simulink library "halout"  (R2021b)
settings: Solver=VariableStepAuto  StartTime=0.0  StopTime=10.0  RelTol=1e-3
undefined symbols (not defined in the file): C_TASK_5MS_S, FALSE, KHAL_CAN1TxReq_flg, KHAL_CAN2TxReq_flg, KHAL_CAN3FD3VCU1toNIDECTxReq_flg, KHAL_CAN3FD3VCU1TxReq_flg, KHAL_CAN3FD3VCU2E2E_flg, KHAL_CAN3FD3VCU2toNIDECE2E_flg, KHAL_CAN3FD3VCU2toNIDECTxReq_flg, KHAL_CAN3FD3VCU2TxReq_flg, KHAL_CAN3TxReq_flg, KHAL_CAN4FD4CE1000E2E_flg, KHAL_CAN4FD4CE1000TxReq_flg, KHAL_CAN4TxReq_flg, KHAL_CAN5TxReq_flg, KHAL_CAN7TxReq_flg, ONE_INT, TRUE, ZERO_INT
libraries: FVT_lib x258, simulink x115
(part 8 of 17)

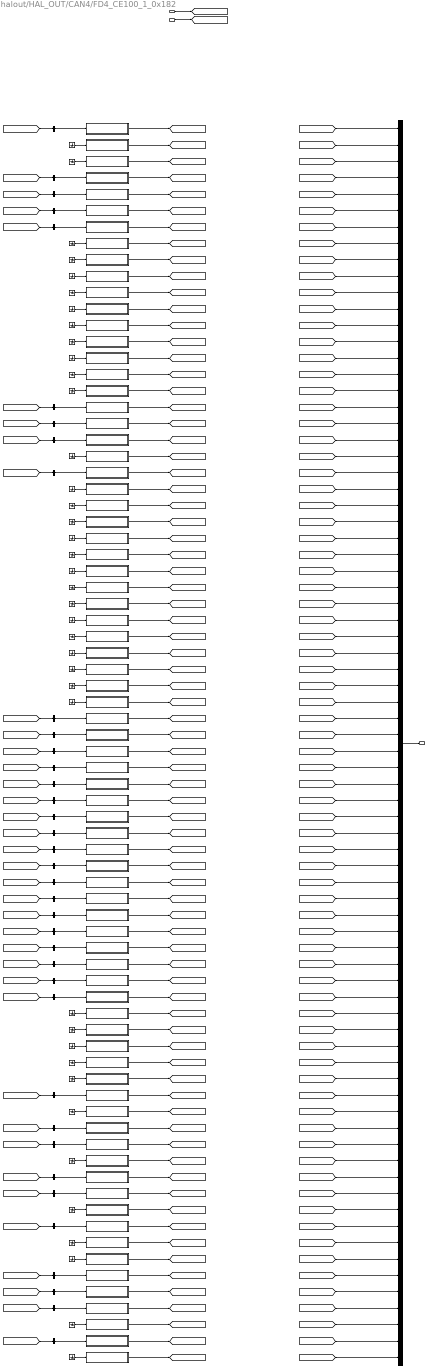
== system halout/HAL_OUT/CAN4/FD4_CE100_1_0x182 ==
  BSCP_outputs : Inport  OutDataTypeStr=Bus: BSCP_outputs
  BOUTP_outputs : Inport  Port=2  OutDataTypeStr=Bus: BOUTP_outputs
  ACSubMode : Subsystem
  APTCActFrRiPwr : Subsystem
  BatLoopActWtFlw : Subsystem
  BatteryMode : Subsystem
  CCUACLampSts : Subsystem
  CCUACMaxLampSts : Subsystem
  CCUAutoLampSts : Subsystem
  CCUAutoMidLampSts : Subsystem
  CCUCbnPreACWkSts : Subsystem
  CCUCbnPreEstimdTi : Subsystem
  CCUCbnPreSts : Subsystem
  CCUDispalyRequest : Subsystem
  CCUEcoSts : Subsystem
  CCUFrtOnOffLampSts : Subsystem
  CCUHEATMaxLampSts : Subsystem
  CCUHiVoltageReq : Subsystem
  CCURrOnOffLampSts : Subsystem
  CCUSyncLampSts : Subsystem
  CabinMode : Subsystem
  CoolgFanActDuty : Subsystem
  DeiceModReq : Subsystem
  EDriveMode : Subsystem
  FDBlowerCmd : Subsystem
  FDCTHCMCLEVentYSta : Subsystem
  FDCTHCMCLEVentZSta : Subsystem
  FDCTHCMCLVentSta : Subsystem
  FDCTHCMCREVentYSta : Subsystem
  FDCTHCMCREVentZSta : Subsystem
  FDCTHCMCRVentSta : Subsystem
  FDCTHCMDrEVentModeSta : Subsystem
  FDCTHCMDrEVentYSta : Subsystem
  FDCTHCMDrEVentZSta : Subsystem
  FDCTHCMDrVentSta : Subsystem
  FDCTHCMPsEVentModeSta : Subsystem
  FDCTHCMPsEVentYSta : Subsystem
  FDCTHCMPsEVentZSta : Subsystem
  FDCTHCMPsVentSta : Subsystem
  FDCompCmd : Subsystem
  FDEWP1Cmd : Subsystem
  FDEWP2Cmd : Subsystem
  FDEWP3Cmd : Subsystem
  FDEXV1Cmd : Subsystem
  FDEXV2Cmd : Subsystem
  FDFWVCmd : Subsystem
  FDFrLeAPTCHeatPwrCmd : Subsystem
  FDFrRiAPTCHeatPwrCmd : Subsystem
  FDFrWPTCHeatPwrCmd : Subsystem
  FDRecyAutoCmd : Subsystem
  FDRrAPTCHeatPwrCmd : Subsystem
  FDSOTXVCmd : Subsystem
  FDSOV1Cmd : Subsystem
  FDSOV2Cmd : Subsystem
  FDSOV3Cmd : Subsystem
  FDTWVCmd : Subsystem
  FrCoolantflow : Subsystem
  FrCoolanttemp : Subsystem
  Ground{,1..38} (39 alike) : Ground
  HPThermalRecoveryReq : Subsystem
  RrCoolantflow : Subsystem
  RrCoolanttemp : Subsystem
  bus_creator : BusCreator  Inputs=76  OutDataTypeStr=Bus: DT_CAN4_SG_FD4_CE100_1  NonVirtualBus=on
  bus_selector : BusSelector  OutputSignals=VOUTP_ACSubMode_enum
  bus_selector1 : BusSelector  OutputSignals=VOUTP_BatteryMode_enum
  bus_selector10 : BusSelector  OutputSignals=VOUTP_FDCompCmd_rpm
  bus_selector11 : BusSelector  OutputSignals=VOUTP_FDEWP1Cmd_enum
  bus_selector12 : BusSelector  OutputSignals=VOUTP_FDEWP2Cmd_enum
  bus_selector13 : BusSelector  OutputSignals=VOUTP_FDEWP3Cmd_enum
  bus_selector14 : BusSelector  OutputSignals=VOUTP_FDEXV1Cmd_step
  bus_selector15 : BusSelector  OutputSignals=VOUTP_FDEXV2Cmd_step
  bus_selector16 : BusSelector  OutputSignals=VOUTP_FDFWVCmd_flg
  bus_selector17 : BusSelector  OutputSignals=VOUTP_FDFrLeAPTCHeatPwrCmd_W
  bus_selector18 : BusSelector  OutputSignals=VOUTP_FDFrRiAPTCHeatPwrCmd_W
  bus_selector19 : BusSelector  OutputSignals=VOUTP_FDFrWPTCHeatPwrCmd_W
  bus_selector2 : BusSelector  OutputSignals=VOUTP_CCUACLampSts_flg
  bus_selector20 : BusSelector  OutputSignals=VOUTP_FDRecyAutoCmd_enum
  bus_selector21 : BusSelector  OutputSignals=VOUTP_FDRrAPTCHeatPwrCmd_W
  bus_selector22 : BusSelector  OutputSignals=VOUTP_FDSOTXVCmd_flg
  bus_selector23 : BusSelector  OutputSignals=VOUTP_FDSOV1Cmd_flg
  bus_selector24 : BusSelector  OutputSignals=VOUTP_FDSOV2Cmd_flg
  bus_selector25 : BusSelector  OutputSignals=VOUTP_FDSOV3Cmd_flg
  bus_selector26 : BusSelector  OutputSignals=VOUTP_FDTWVCmd_pct
  bus_selector27 : BusSelector  OutputSignals=VOUTP_sigAirIntenZon1St_enum
  bus_selector28 : BusSelector  OutputSignals=VOUTP_sigAmbAirT_C
  bus_selector29 : BusSelector  OutputSignals=VOUTP_sigCbnAirT_C
  bus_selector3 : BusSelector  OutputSignals=VOUTP_CCUACMaxLampSts_flg
  bus_selector30 : BusSelector  OutputSignals=VOUTP_sigCbnSolarLeft_W
  bus_selector31 : BusSelector  OutputSignals=VOUTP_sigCbnSolarRight_W
  bus_selector32 : BusSelector  OutputSignals=VOUTP_sigClntTHvBattOut_C
  bus_selector33 : BusSelector  OutputSignals=VOUTP_sigRecircSt_flg
  bus_selector34 : BusSelector  OutputSignals=VOUTP_sigSetTempZon1St_C
  bus_selector35 : BusSelector  OutputSignals=VOUTP_sigSetTempZon2St_C
  bus_selector36 : BusSelector  OutputSignals=VOUTP_sigWindDirZon1St_enum
  bus_selector4 : BusSelector  OutputSignals=VOUTP_CCUAutoLampSts_flg
  bus_selector5 : BusSelector  OutputSignals=VOUTP_CCUSyncLampSts_flg
  bus_selector6 : BusSelector  OutputSignals=VOUTP_CabinMode_enum
  bus_selector7 : BusSelector  OutputSignals=VOUTP_CoolgFanActDuty_pct
  bus_selector8 : BusSelector  OutputSignals=VOUTP_EDriveMode_enum
  bus_selector9 : BusSelector  OutputSignals=VOUTP_FDBlowerCmd_pct
  sigAirIntenZon1St : Subsystem
  sigAirIntenZon3St : Subsystem
  sigAmbAirT : Subsystem
  sigCbnAirT : Subsystem
  sigCbnPTCPwrAct : Subsystem
  sigCbnSolarLeft : Subsystem
  sigCbnSolarRight : Subsystem
  sigClmtCmprPwrAct : Subsystem
  sigClntTHvBattOut : Subsystem
  sigDfrstSt : Subsystem
  sigHvacSt : Subsystem
  sigRecircSt : Subsystem
  sigSetTempZon1St : Subsystem
  sigSetTempZon2St : Subsystem
  sigSetTempZon3St : Subsystem
  sigWindDirZon1St : Subsystem
  sigWindDirZon3St : Subsystem
  FD4_CE100_1 : Outport
  wires:
  BSCP_outputs/1 -> [BSCP_outputs]
  BOUTP_outputs/1 -> [BOUTP_outputs]
  [CAN4_ACSubMode] -> bus_creator/1  "CAN4_ACSubMode"
  [CAN4_APTC_ActFrRiPwr] -> bus_creator/2  "CAN4_APTC_ActFrRiPwr"
  [CAN4_BatLoopActWtFlw] -> bus_creator/3  "CAN4_BatLoopActWtFlw"
  [CAN4_BatteryMode] -> bus_creator/4  "CAN4_BatteryMode"
  [CAN4_CCU_ACLampSts] -> bus_creator/5  "CAN4_CCU_ACLampSts"
  [CAN4_CCU_ACMaxLampSts] -> bus_creator/6  "CAN4_CCU_ACMaxLampSts"
  [CAN4_CCU_AutoLampSts] -> bus_creator/7  "CAN4_CCU_AutoLampSts"
  [CAN4_CCU_AutoMidLampSts] -> bus_creator/8  "CAN4_CCU_AutoMidLampSts"
  [CAN4_CCU_CbnPreACWkSts] -> bus_creator/9  "CAN4_CCU_CbnPreACWkSts"
  [CAN4_CCU_CbnPreEstimdTi] -> bus_creator/10  "CAN4_CCU_CbnPreEstimdTi"
  [CAN4_CCU_CbnPreSts] -> bus_creator/11  "CAN4_CCU_CbnPreSts"
  [CAN4_CCU_Dispaly_Request] -> bus_creator/12  "CAN4_CCU_Dispaly_Request"
  [CAN4_CCU_EcoSts] -> bus_creator/13  "CAN4_CCU_EcoSts"
  [CAN4_CCU_FrtOnOffLampSts] -> bus_creator/14  "CAN4_CCU_FrtOnOffLampSts"
  [CAN4_CCU_HEATMaxLampSts] -> bus_creator/15  "CAN4_CCU_HEATMaxLampSts"
  [CAN4_CCU_HiVoltageReq] -> bus_creator/16  "CAN4_CCU_HiVoltageReq"
  [CAN4_CCU_RrOnOffLampSts] -> bus_creator/17  "CAN4_CCU_RrOnOffLampSts"
  [CAN4_CCU_SyncLampSts] -> bus_creator/18  "CAN4_CCU_SyncLampSts"
  [CAN4_CabinMode] -> bus_creator/19  "CAN4_CabinMode"
  [CAN4_CoolgFanActDuty] -> bus_creator/20  "CAN4_CoolgFanActDuty"
  [CAN4_DeiceModReq] -> bus_creator/21  "CAN4_DeiceModReq"
  [CAN4_EDriveMode] -> bus_creator/22  "CAN4_EDriveMode"
  [CAN4_FDC_THCM_CLEVentY_Sta] -> bus_creator/23  "CAN4_FDC_THCM_CLEVentY_Sta"
  [CAN4_FDC_THCM_CLEVentZ_Sta] -> bus_creator/24  "CAN4_FDC_THCM_CLEVentZ_Sta"
  [CAN4_FDC_THCM_CLVent_Sta] -> bus_creator/25  "CAN4_FDC_THCM_CLVent_Sta"
  [CAN4_FDC_THCM_CREVentY_Sta] -> bus_creator/26  "CAN4_FDC_THCM_CREVentY_Sta"
  [CAN4_FDC_THCM_CREVentZ_Sta] -> bus_creator/27  "CAN4_FDC_THCM_CREVentZ_Sta"
  [CAN4_FDC_THCM_CRVent_Sta] -> bus_creator/28  "CAN4_FDC_THCM_CRVent_Sta"
  [CAN4_FDC_THCM_DrEVentMode_Sta] -> bus_creator/29  "CAN4_FDC_THCM_DrEVentMode_Sta"
  [CAN4_FDC_THCM_DrEVentY_Sta] -> bus_creator/30  "CAN4_FDC_THCM_DrEVentY_Sta"
  [CAN4_FDC_THCM_DrEVentZ_Sta] -> bus_creator/31  "CAN4_FDC_THCM_DrEVentZ_Sta"
  [CAN4_FDC_THCM_DrVent_Sta] -> bus_creator/32  "CAN4_FDC_THCM_DrVent_Sta"
  [CAN4_FDC_THCM_PsEVentMode_Sta] -> bus_creator/33  "CAN4_FDC_THCM_PsEVentMode_Sta"
  [CAN4_FDC_THCM_PsEVentY_Sta] -> bus_creator/34  "CAN4_FDC_THCM_PsEVentY_Sta"
  [CAN4_FDC_THCM_PsEVentZ_Sta] -> bus_creator/35  "CAN4_FDC_THCM_PsEVentZ_Sta"
  [CAN4_FDC_THCM_PsVent_Sta] -> bus_creator/36  "CAN4_FDC_THCM_PsVent_Sta"
  [CAN4_FD_Blower_Cmd] -> bus_creator/37  "CAN4_FD_Blower_Cmd"
  [CAN4_FD_Comp_Cmd] -> bus_creator/38  "CAN4_FD_Comp_Cmd"
  [CAN4_FD_EWP1_Cmd] -> bus_creator/39  "CAN4_FD_EWP1_Cmd"
  [CAN4_FD_EWP2_Cmd] -> bus_creator/40  "CAN4_FD_EWP2_Cmd"
  [CAN4_FD_EWP3_Cmd] -> bus_creator/41  "CAN4_FD_EWP3_Cmd"
  [CAN4_FD_EXV1_Cmd] -> bus_creator/42  "CAN4_FD_EXV1_Cmd"
  [CAN4_FD_EXV2_Cmd] -> bus_creator/43  "CAN4_FD_EXV2_Cmd"
  [CAN4_FD_FWV_Cmd] -> bus_creator/44  "CAN4_FD_FWV_Cmd"
  [CAN4_FD_FrLeAPTCHeatPwr_Cmd] -> bus_creator/45  "CAN4_FD_FrLeAPTCHeatPwr_Cmd"
  [CAN4_FD_FrRiAPTCHeatPwr_Cmd] -> bus_creator/46  "CAN4_FD_FrRiAPTCHeatPwr_Cmd"
  [CAN4_FD_FrWPTCHeatPwr_Cmd] -> bus_creator/47  "CAN4_FD_FrWPTCHeatPwr_Cmd"
  [CAN4_FD_RecyAuto_Cmd] -> bus_creator/48  "CAN4_FD_RecyAuto_Cmd"
  [CAN4_FD_RrAPTCHeatPwr_Cmd] -> bus_creator/49  "CAN4_FD_RrAPTCHeatPwr_Cmd"
  [CAN4_FD_SOTXV_Cmd] -> bus_creator/50  "CAN4_FD_SOTXV_Cmd"
  [CAN4_FD_SOV1_Cmd] -> bus_creator/51  "CAN4_FD_SOV1_Cmd"
  [CAN4_FD_SOV2_Cmd] -> bus_creator/52  "CAN4_FD_SOV2_Cmd"
  [CAN4_FD_SOV3_Cmd] -> bus_creator/53  "CAN4_FD_SOV3_Cmd"
  [CAN4_FD_TWV_Cmd] -> bus_creator/54  "CAN4_FD_TWV_Cmd"
  [CAN4_Fr_Coolantflow] -> bus_creator/55  "CAN4_Fr_Coolantflow"
  [CAN4_Fr_Coolanttemp] -> bus_creator/56  "CAN4_Fr_Coolanttemp"
  [CAN4_HPThermalRecoveryReq] -> bus_creator/57  "CAN4_HPThermalRecoveryReq"
  [CAN4_Rr_Coolantflow] -> bus_creator/58  "CAN4_Rr_Coolantflow"
  [CAN4_Rr_Coolanttemp] -> bus_creator/59  "CAN4_Rr_Coolanttemp"
  [CAN4_sigAirIntenZon1St] -> bus_creator/60  "CAN4_sigAirIntenZon1St"
  [CAN4_sigAirIntenZon3St] -> bus_creator/61  "CAN4_sigAirIntenZon3St"
  [CAN4_sigAmbAirT] -> bus_creator/62  "CAN4_sigAmbAirT"
  [CAN4_sigCbnAirT] -> bus_creator/63  "CAN4_sigCbnAirT"
  [CAN4_sigCbnPTCPwrAct] -> bus_creator/64  "CAN4_sigCbnPTCPwrAct"
  [CAN4_sigCbnSolarLeft] -> bus_creator/65  "CAN4_sigCbnSolarLeft"
  [CAN4_sigCbnSolarRight] -> bus_creator/66  "CAN4_sigCbnSolarRight"
  [CAN4_sigClmtCmprPwrAct] -> bus_creator/67  "CAN4_sigClmtCmprPwrAct"
  [CAN4_sigClntTHvBattOut] -> bus_creator/68  "CAN4_sigClntTHvBattOut"
  [CAN4_sigDfrstSt] -> bus_creator/69  "CAN4_sigDfrstSt"
  [CAN4_sigHvacSt] -> bus_creator/70  "CAN4_sigHvacSt"
  [CAN4_sigRecircSt] -> bus_creator/71  "CAN4_sigRecircSt"
  [CAN4_sigSetTempZon1St] -> bus_creator/72  "CAN4_sigSetTempZon1St"
  [CAN4_sigSetTempZon2St] -> bus_creator/73  "CAN4_sigSetTempZon2St"
  [CAN4_sigSetTempZon3St] -> bus_creator/74  "CAN4_sigSetTempZon3St"
  [CAN4_sigWindDirZon1St] -> bus_creator/75  "CAN4_sigWindDirZon1St"
  [CAN4_sigWindDirZon3St] -> bus_creator/76  "CAN4_sigWindDirZon3St"
  bus_creator/1 -> FD4_CE100_1/1
  ACSubMode/1(CAN4_ACSubMode) -> [CAN4_ACSubMode]
  APTCActFrRiPwr/1(CAN4_APTC_ActFrRiPwr) -> [CAN4_APTC_ActFrRiPwr]
  BatLoopActWtFlw/1(CAN4_BatLoopActWtFlw) -> [CAN4_BatLoopActWtFlw]
  BatteryMode/1(CAN4_BatteryMode) -> [CAN4_BatteryMode]
  CCUACLampSts/1(CAN4_CCU_ACLampSts) -> [CAN4_CCU_ACLampSts]
  CCUACMaxLampSts/1(CAN4_CCU_ACMaxLampSts) -> [CAN4_CCU_ACMaxLampSts]
  CCUAutoLampSts/1(CAN4_CCU_AutoLampSts) -> [CAN4_CCU_AutoLampSts]
  CCUAutoMidLampSts/1(CAN4_CCU_AutoMidLampSts) -> [CAN4_CCU_AutoMidLampSts]
  CCUCbnPreACWkSts/1(CAN4_CCU_CbnPreACWkSts) -> [CAN4_CCU_CbnPreACWkSts]
  CCUCbnPreEstimdTi/1(CAN4_CCU_CbnPreEstimdTi) -> [CAN4_CCU_CbnPreEstimdTi]
  CCUCbnPreSts/1(CAN4_CCU_CbnPreSts) -> [CAN4_CCU_CbnPreSts]
  CCUDispalyRequest/1(CAN4_CCU_Dispaly_Request) -> [CAN4_CCU_Dispaly_Request]
  CCUEcoSts/1(CAN4_CCU_EcoSts) -> [CAN4_CCU_EcoSts]
  CCUFrtOnOffLampSts/1(CAN4_CCU_FrtOnOffLampSts) -> [CAN4_CCU_FrtOnOffLampSts]
  CCUHEATMaxLampSts/1(CAN4_CCU_HEATMaxLampSts) -> [CAN4_CCU_HEATMaxLampSts]
  CCUHiVoltageReq/1(CAN4_CCU_HiVoltageReq) -> [CAN4_CCU_HiVoltageReq]
  CCURrOnOffLampSts/1(CAN4_CCU_RrOnOffLampSts) -> [CAN4_CCU_RrOnOffLampSts]
  CCUSyncLampSts/1(CAN4_CCU_SyncLampSts) -> [CAN4_CCU_SyncLampSts]
  CabinMode/1(CAN4_CabinMode) -> [CAN4_CabinMode]
  CoolgFanActDuty/1(CAN4_CoolgFanActDuty) -> [CAN4_CoolgFanActDuty]
  DeiceModReq/1(CAN4_DeiceModReq) -> [CAN4_DeiceModReq]
  EDriveMode/1(CAN4_EDriveMode) -> [CAN4_EDriveMode]
  FDCTHCMCLEVentYSta/1(CAN4_FDC_THCM_CLEVentY_Sta) -> [CAN4_FDC_THCM_CLEVentY_Sta]
  FDCTHCMCLEVentZSta/1(CAN4_FDC_THCM_CLEVentZ_Sta) -> [CAN4_FDC_THCM_CLEVentZ_Sta]
  FDCTHCMCLVentSta/1(CAN4_FDC_THCM_CLVent_Sta) -> [CAN4_FDC_THCM_CLVent_Sta]
  FDCTHCMCREVentYSta/1(CAN4_FDC_THCM_CREVentY_Sta) -> [CAN4_FDC_THCM_CREVentY_Sta]
  FDCTHCMCREVentZSta/1(CAN4_FDC_THCM_CREVentZ_Sta) -> [CAN4_FDC_THCM_CREVentZ_Sta]
  FDCTHCMCRVentSta/1(CAN4_FDC_THCM_CRVent_Sta) -> [CAN4_FDC_THCM_CRVent_Sta]
  FDCTHCMDrEVentModeSta/1(CAN4_FDC_THCM_DrEVentMode_Sta) -> [CAN4_FDC_THCM_DrEVentMode_Sta]
  FDCTHCMDrEVentYSta/1(CAN4_FDC_THCM_DrEVentY_Sta) -> [CAN4_FDC_THCM_DrEVentY_Sta]
  FDCTHCMDrEVentZSta/1(CAN4_FDC_THCM_DrEVentZ_Sta) -> [CAN4_FDC_THCM_DrEVentZ_Sta]
  FDCTHCMDrVentSta/1(CAN4_FDC_THCM_DrVent_Sta) -> [CAN4_FDC_THCM_DrVent_Sta]
  FDCTHCMPsEVentModeSta/1(CAN4_FDC_THCM_PsEVentMode_Sta) -> [CAN4_FDC_THCM_PsEVentMode_Sta]
  FDCTHCMPsEVentYSta/1(CAN4_FDC_THCM_PsEVentY_Sta) -> [CAN4_FDC_THCM_PsEVentY_Sta]
  FDCTHCMPsEVentZSta/1(CAN4_FDC_THCM_PsEVentZ_Sta) -> [CAN4_FDC_THCM_PsEVentZ_Sta]
  FDCTHCMPsVentSta/1(CAN4_FDC_THCM_PsVent_Sta) -> [CAN4_FDC_THCM_PsVent_Sta]
  FDBlowerCmd/1(CAN4_FD_Blower_Cmd) -> [CAN4_FD_Blower_Cmd]
  FDCompCmd/1(CAN4_FD_Comp_Cmd) -> [CAN4_FD_Comp_Cmd]
  FDEWP1Cmd/1(CAN4_FD_EWP1_Cmd) -> [CAN4_FD_EWP1_Cmd]
  FDEWP2Cmd/1(CAN4_FD_EWP2_Cmd) -> [CAN4_FD_EWP2_Cmd]
  FDEWP3Cmd/1(CAN4_FD_EWP3_Cmd) -> [CAN4_FD_EWP3_Cmd]
  FDEXV1Cmd/1(CAN4_FD_EXV1_Cmd) -> [CAN4_FD_EXV1_Cmd]
  FDEXV2Cmd/1(CAN4_FD_EXV2_Cmd) -> [CAN4_FD_EXV2_Cmd]
  FDFWVCmd/1(CAN4_FD_FWV_Cmd) -> [CAN4_FD_FWV_Cmd]
  FDFrLeAPTCHeatPwrCmd/1(CAN4_FD_FrLeAPTCHeatPwr_Cmd) -> [CAN4_FD_FrLeAPTCHeatPwr_Cmd]
  FDFrRiAPTCHeatPwrCmd/1(CAN4_FD_FrRiAPTCHeatPwr_Cmd) -> [CAN4_FD_FrRiAPTCHeatPwr_Cmd]
  FDFrWPTCHeatPwrCmd/1(CAN4_FD_FrWPTCHeatPwr_Cmd) -> [CAN4_FD_FrWPTCHeatPwr_Cmd]
  FDRecyAutoCmd/1(CAN4_FD_RecyAuto_Cmd) -> [CAN4_FD_RecyAuto_Cmd]
  FDRrAPTCHeatPwrCmd/1(CAN4_FD_RrAPTCHeatPwr_Cmd) -> [CAN4_FD_RrAPTCHeatPwr_Cmd]
  FDSOTXVCmd/1(CAN4_FD_SOTXV_Cmd) -> [CAN4_FD_SOTXV_Cmd]
  FDSOV1Cmd/1(CAN4_FD_SOV1_Cmd) -> [CAN4_FD_SOV1_Cmd]
  FDSOV2Cmd/1(CAN4_FD_SOV2_Cmd) -> [CAN4_FD_SOV2_Cmd]
  FDSOV3Cmd/1(CAN4_FD_SOV3_Cmd) -> [CAN4_FD_SOV3_Cmd]
  FDTWVCmd/1(CAN4_FD_TWV_Cmd) -> [CAN4_FD_TWV_Cmd]
  FrCoolantflow/1(CAN4_Fr_Coolantflow) -> [CAN4_Fr_Coolantflow]
  FrCoolanttemp/1(CAN4_Fr_Coolanttemp) -> [CAN4_Fr_Coolanttemp]
  HPThermalRecoveryReq/1(CAN4_HPThermalRecoveryReq) -> [CAN4_HPThermalRecoveryReq]
  RrCoolantflow/1(CAN4_Rr_Coolantflow) -> [CAN4_Rr_Coolantflow]
  RrCoolanttemp/1(CAN4_Rr_Coolanttemp) -> [CAN4_Rr_Coolanttemp]
  sigAirIntenZon1St/1(CAN4_sigAirIntenZon1St) -> [CAN4_sigAirIntenZon1St]
  sigAirIntenZon3St/1(CAN4_sigAirIntenZon3St) -> [CAN4_sigAirIntenZon3St]
  sigAmbAirT/1(CAN4_sigAmbAirT) -> [CAN4_sigAmbAirT]
  sigCbnAirT/1(CAN4_sigCbnAirT) -> [CAN4_sigCbnAirT]
  sigCbnPTCPwrAct/1(CAN4_sigCbnPTCPwrAct) -> [CAN4_sigCbnPTCPwrAct]
  sigCbnSolarLeft/1(CAN4_sigCbnSolarLeft) -> [CAN4_sigCbnSolarLeft]
  sigCbnSolarRight/1(CAN4_sigCbnSolarRight) -> [CAN4_sigCbnSolarRight]
  sigClmtCmprPwrAct/1(CAN4_sigClmtCmprPwrAct) -> [CAN4_sigClmtCmprPwrAct]
  sigClntTHvBattOut/1(CAN4_sigClntTHvBattOut) -> [CAN4_sigClntTHvBattOut]
  sigDfrstSt/1(CAN4_sigDfrstSt) -> [CAN4_sigDfrstSt]
  sigHvacSt/1(CAN4_sigHvacSt) -> [CAN4_sigHvacSt]
  sigRecircSt/1(CAN4_sigRecircSt) -> [CAN4_sigRecircSt]
  sigSetTempZon1St/1(CAN4_sigSetTempZon1St) -> [CAN4_sigSetTempZon1St]
  sigSetTempZon2St/1(CAN4_sigSetTempZon2St) -> [CAN4_sigSetTempZon2St]
  sigSetTempZon3St/1(CAN4_sigSetTempZon3St) -> [CAN4_sigSetTempZon3St]
  sigWindDirZon1St/1(CAN4_sigWindDirZon1St) -> [CAN4_sigWindDirZon1St]
  sigWindDirZon3St/1(CAN4_sigWindDirZon3St) -> [CAN4_sigWindDirZon3St]
  bus_selector/1 -> ACSubMode/1(ACSubMode)  "<VOUTP_ACSubMode_enum>"
  [BOUTP_outputs] -> bus_selector/1
  Ground/1 -> APTCActFrRiPwr/1(APTCActFrRiPwr)
  Ground1/1 -> BatLoopActWtFlw/1(BatLoopActWtFlw)
  bus_selector1/1 -> BatteryMode/1(BatteryMode)  "<VOUTP_BatteryMode_enum>"
  [BOUTP_outputs] -> bus_selector1/1
  bus_selector2/1 -> CCUACLampSts/1(CCUACLampSts)  "<VOUTP_CCUACLampSts_flg>"
  [BOUTP_outputs] -> bus_selector2/1
  bus_selector3/1 -> CCUACMaxLampSts/1(CCUACMaxLampSts)  "<VOUTP_CCUACMaxLampSts_flg>"
  [BOUTP_outputs] -> bus_selector3/1
  bus_selector4/1 -> CCUAutoLampSts/1(CCUAutoLampSts)  "<VOUTP_CCUAutoLampSts_flg>"
  [BOUTP_outputs] -> bus_selector4/1
  Ground2/1 -> CCUAutoMidLampSts/1(CCUAutoMidLampSts)
  Ground3/1 -> CCUCbnPreACWkSts/1(CCUCbnPreACWkSts)
  Ground4/1 -> CCUCbnPreEstimdTi/1(CCUCbnPreEstimdTi)
  Ground5/1 -> CCUCbnPreSts/1(CCUCbnPreSts)
  Ground6/1 -> CCUDispalyRequest/1(CCUDispalyRequest)
  Ground7/1 -> CCUEcoSts/1(CCUEcoSts)
  Ground8/1 -> CCUFrtOnOffLampSts/1(CCUFrtOnOffLampSts)
  Ground9/1 -> CCUHEATMaxLampSts/1(CCUHEATMaxLampSts)
  Ground10/1 -> CCUHiVoltageReq/1(CCUHiVoltageReq)
  Ground11/1 -> CCURrOnOffLampSts/1(CCURrOnOffLampSts)
  bus_selector5/1 -> CCUSyncLampSts/1(CCUSyncLampSts)  "<VOUTP_CCUSyncLampSts_flg>"
  [BOUTP_outputs] -> bus_selector5/1
  bus_selector6/1 -> CabinMode/1(CabinMode)  "<VOUTP_CabinMode_enum>"
  [BOUTP_outputs] -> bus_selector6/1
  bus_selector7/1 -> CoolgFanActDuty/1(CoolgFanActDuty)  "<VOUTP_CoolgFanActDuty_pct>"
  [BOUTP_outputs] -> bus_selector7/1
  Ground12/1 -> DeiceModReq/1(DeiceModReq)
  bus_selector8/1 -> EDriveMode/1(EDriveMode)  "<VOUTP_EDriveMode_enum>"
  [BOUTP_outputs] -> bus_selector8/1
  Ground13/1 -> FDCTHCMCLEVentYSta/1(FDCTHCMCLEVentYSta)
  Ground14/1 -> FDCTHCMCLEVentZSta/1(FDCTHCMCLEVentZSta)
  Ground15/1 -> FDCTHCMCLVentSta/1(FDCTHCMCLVentSta)
  Ground16/1 -> FDCTHCMCREVentYSta/1(FDCTHCMCREVentYSta)
  Ground17/1 -> FDCTHCMCREVentZSta/1(FDCTHCMCREVentZSta)
  Ground18/1 -> FDCTHCMCRVentSta/1(FDCTHCMCRVentSta)
  Ground19/1 -> FDCTHCMDrEVentModeSta/1(FDCTHCMDrEVentModeSta)
  Ground20/1 -> FDCTHCMDrEVentYSta/1(FDCTHCMDrEVentYSta)
  Ground21/1 -> FDCTHCMDrEVentZSta/1(FDCTHCMDrEVentZSta)
  Ground22/1 -> FDCTHCMDrVentSta/1(FDCTHCMDrVentSta)
  Ground23/1 -> FDCTHCMPsEVentModeSta/1(FDCTHCMPsEVentModeSta)
  Ground24/1 -> FDCTHCMPsEVentYSta/1(FDCTHCMPsEVentYSta)
  Ground25/1 -> FDCTHCMPsEVentZSta/1(FDCTHCMPsEVentZSta)
  Ground26/1 -> FDCTHCMPsVentSta/1(FDCTHCMPsVentSta)
  bus_selector9/1 -> FDBlowerCmd/1(FDBlowerCmd)  "<VOUTP_FDBlowerCmd_pct>"
  [BOUTP_outputs] -> bus_selector9/1
  bus_selector10/1 -> FDCompCmd/1(FDCompCmd)  "<VOUTP_FDCompCmd_rpm>"
  [BOUTP_outputs] -> bus_selector10/1
  bus_selector11/1 -> FDEWP1Cmd/1(FDEWP1Cmd)  "<VOUTP_FDEWP1Cmd_enum>"
  [BOUTP_outputs] -> bus_selector11/1
  bus_selector12/1 -> FDEWP2Cmd/1(FDEWP2Cmd)  "<VOUTP_FDEWP2Cmd_enum>"
  [BOUTP_outputs] -> bus_selector12/1
  bus_selector13/1 -> FDEWP3Cmd/1(FDEWP3Cmd)  "<VOUTP_FDEWP3Cmd_enum>"
  [BOUTP_outputs] -> bus_selector13/1
  bus_selector14/1 -> FDEXV1Cmd/1(FDEXV1Cmd)  "<VOUTP_FDEXV1Cmd_step>"
  [BOUTP_outputs] -> bus_selector14/1
  bus_selector15/1 -> FDEXV2Cmd/1(FDEXV2Cmd)  "<VOUTP_FDEXV2Cmd_step>"
  [BOUTP_outputs] -> bus_selector15/1
  bus_selector16/1 -> FDFWVCmd/1(FDFWVCmd)  "<VOUTP_FDFWVCmd_flg>"
  [BOUTP_outputs] -> bus_selector16/1
  bus_selector17/1 -> FDFrLeAPTCHeatPwrCmd/1(FDFrLeAPTCHeatPwrCmd)  "<VOUTP_FDFrLeAPTCHeatPwrCmd_W>"
  [BOUTP_outputs] -> bus_selector17/1
  bus_selector18/1 -> FDFrRiAPTCHeatPwrCmd/1(FDFrRiAPTCHeatPwrCmd)  "<VOUTP_FDFrRiAPTCHeatPwrCmd_W>"
  [BOUTP_outputs] -> bus_selector18/1
  bus_selector19/1 -> FDFrWPTCHeatPwrCmd/1(FDFrWPTCHeatPwrCmd)  "<VOUTP_FDFrWPTCHeatPwrCmd_W>"
  [BOUTP_outputs] -> bus_selector19/1
  bus_selector20/1 -> FDRecyAutoCmd/1(FDRecyAutoCmd)  "<VOUTP_FDRecyAutoCmd_enum>"
  [BOUTP_outputs] -> bus_selector20/1
  bus_selector21/1 -> FDRrAPTCHeatPwrCmd/1(FDRrAPTCHeatPwrCmd)  "<VOUTP_FDRrAPTCHeatPwrCmd_W>"
  [BOUTP_outputs] -> bus_selector21/1
  bus_selector22/1 -> FDSOTXVCmd/1(FDSOTXVCmd)  "<VOUTP_FDSOTXVCmd_flg>"
  [BOUTP_outputs] -> bus_selector22/1
  bus_selector23/1 -> FDSOV1Cmd/1(FDSOV1Cmd)  "<VOUTP_FDSOV1Cmd_flg>"
  [BOUTP_outputs] -> bus_selector23/1
  bus_selector24/1 -> FDSOV2Cmd/1(FDSOV2Cmd)  "<VOUTP_FDSOV2Cmd_flg>"
  [BOUTP_outputs] -> bus_selector24/1
  bus_selector25/1 -> FDSOV3Cmd/1(FDSOV3Cmd)  "<VOUTP_FDSOV3Cmd_flg>"
  [BOUTP_outputs] -> bus_selector25/1
  bus_selector26/1 -> FDTWVCmd/1(FDTWVCmd)  "<VOUTP_FDTWVCmd_pct>"
  [BOUTP_outputs] -> bus_selector26/1
  Ground27/1 -> FrCoolantflow/1(FrCoolantflow)
  Ground28/1 -> FrCoolanttemp/1(FrCoolanttemp)
  Ground29/1 -> HPThermalRecoveryReq/1(HPThermalRecoveryReq)
  Ground30/1 -> RrCoolantflow/1(RrCoolantflow)
  Ground31/1 -> RrCoolanttemp/1(RrCoolanttemp)
  bus_selector27/1 -> sigAirIntenZon1St/1(sigAirIntenZon1St)  "<VOUTP_sigAirIntenZon1St_enum>"
  [BOUTP_outputs] -> bus_selector27/1
  Ground32/1 -> sigAirIntenZon3St/1(sigAirIntenZon3St)
  bus_selector28/1 -> sigAmbAirT/1(sigAmbAirT)  "<VOUTP_sigAmbAirT_C>"
  [BOUTP_outputs] -> bus_selector28/1
  bus_selector29/1 -> sigCbnAirT/1(sigCbnAirT)  "<VOUTP_sigCbnAirT_C>"
  [BOUTP_outputs] -> bus_selector29/1
  Ground33/1 -> sigCbnPTCPwrAct/1(sigCbnPTCPwrAct)
  bus_selector30/1 -> sigCbnSolarLeft/1(sigCbnSolarLeft)  "<VOUTP_sigCbnSolarLeft_W>"
  [BOUTP_outputs] -> bus_selector30/1
  bus_selector31/1 -> sigCbnSolarRight/1(sigCbnSolarRight)  "<VOUTP_sigCbnSolarRight_W>"
  [BOUTP_outputs] -> bus_selector31/1
  Ground34/1 -> sigClmtCmprPwrAct/1(sigClmtCmprPwrAct)
  bus_selector32/1 -> sigClntTHvBattOut/1(sigClntTHvBattOut)  "<VOUTP_sigClntTHvBattOut_C>"
  [BOUTP_outputs] -> bus_selector32/1
  Ground35/1 -> sigDfrstSt/1(sigDfrstSt)
  Ground36/1 -> sigHvacSt/1(sigHvacSt)
  bus_selector33/1 -> sigRecircSt/1(sigRecircSt)  "<VOUTP_sigRecircSt_flg>"
  [BOUTP_outputs] -> bus_selector33/1
  bus_selector34/1 -> sigSetTempZon1St/1(sigSetTempZon1St)  "<VOUTP_sigSetTempZon1St_C>"
  [BOUTP_outputs] -> bus_selector34/1
  bus_selector35/1 -> sigSetTempZon2St/1(sigSetTempZon2St)  "<VOUTP_sigSetTempZon2St_C>"
  [BOUTP_outputs] -> bus_selector35/1
  Ground37/1 -> sigSetTempZon3St/1(sigSetTempZon3St)
  bus_selector36/1 -> sigWindDirZon1St/1(sigWindDirZon1St)  "<VOUTP_sigWindDirZon1St_enum>"
  [BOUTP_outputs] -> bus_selector36/1
  Ground38/1 -> sigWindDirZon3St/1(sigWindDirZon3St)

== system halout/HAL_OUT/CAN4/FD4_CE100_3_0x201 ==
  BSCP_outputs : Inport  OutDataTypeStr=Bus: BSCP_outputs
  BOUTP_outputs : Inport  Port=2  OutDataTypeStr=Bus: BOUTP_outputs
  FDCBCMBBuzzerCmd : Subsystem
  FDCBCMBBuzzeroutCmd : Subsystem
  FDCBCMEmExitLightCmd : Subsystem
  FDCBCMFrAtmoLampCmd : Subsystem
  FDCBCMFrRmLampBrightCmd : Subsystem
  FDCBCMFrRoomlampCmd : Subsystem
  FDCBCMIBuzzerReqSta : Subsystem
  FDCBCMLSMLPCmd : Subsystem
  FDCBCMLTgateRelCmd : Subsystem
  FDCBCMRSMLPCmd : Subsystem
  FDCBCMRTgateRelCmd : Subsystem
  FDCBCMRevBuzzeroutCmd : Subsystem
  FDCBCMRrAtmoLampCmd : Subsystem
  FDCBCMRrRmLampBrightCmd : Subsystem
  FDCBCMRrRoomlampCmd : Subsystem
  FDCBCMSTurnLpLeftCmd : Subsystem
  FDCBCMSTurnLpRightCmd : Subsystem
  FDCBCMTgateHDSWLSta : Subsystem
  FDCBCMTgateHDSWRSta : Subsystem
  FDCBCMTgateSWLSta : Subsystem
  FDCBCMTgateSWRSta : Subsystem
  FDCBCMTurnLpLActiveCmd : Subsystem
  FDCBCMTurnLpRActiveCmd : Subsystem
  FDCBCMinnerBuzzerCmd : Subsystem
  Ground{,1..9} (10 alike) : Ground
  bus_creator : BusCreator  Inputs=24  OutDataTypeStr=Bus: DT_CAN4_SG_FD4_CE100_3  NonVirtualBus=on
  bus_selector : BusSelector  OutputSignals=VOUTP_BBuzzerCmd_flg
  bus_selector1 : BusSelector  OutputSignals=VOUTP_FrAtmoLampCmd_flg
  bus_selector10 : BusSelector  OutputSignals=VOUTP_TgateSWLSta_flg
  bus_selector11 : BusSelector  OutputSignals=VOUTP_TgateSWRSta_flg
  bus_selector12 : BusSelector  OutputSignals=VOUTP_TurnLpLActiveCmd_flg
  bus_selector13 : BusSelector  OutputSignals=VOUTP_TurnLpRActiveCmd_flg
  bus_selector2 : BusSelector  OutputSignals=VOUTP_LSMLPCmd_flg
  bus_selector3 : BusSelector  OutputSignals=VOUTP_LTgateRelCmd_flg
  bus_selector4 : BusSelector  OutputSignals=VOUTP_RSMLPCmd_flg
  bus_selector5 : BusSelector  OutputSignals=VOUTP_RTgateRelCmd_flg
  bus_selector6 : BusSelector  OutputSignals=VOUTP_RrAtmoLampCmd_flg
  bus_selector7 : BusSelector  OutputSignals=VOUTP_RrRmLampBrightCmd_enum
  bus_selector8 : BusSelector  OutputSignals=VOUTP_TgateHDSWLSta_flg
  bus_selector9 : BusSelector  OutputSignals=VOUTP_TgateHDSWRSta_flg
  FD4_CE100_3 : Outport
  wires:
  BSCP_outputs/1 -> [BSCP_outputs]
  BOUTP_outputs/1 -> [BOUTP_outputs]
  [CAN4_FDC_BCM_BBuzzer_Cmd] -> bus_creator/1  "CAN4_FDC_BCM_BBuzzer_Cmd"
  [CAN4_FDC_BCM_BBuzzerout_Cmd] -> bus_creator/2  "CAN4_FDC_BCM_BBuzzerout_Cmd"
  [CAN4_FDC_BCM_EmExitLight_Cmd] -> bus_creator/3  "CAN4_FDC_BCM_EmExitLight_Cmd"
  [CAN4_FDC_BCM_FrAtmoLamp_Cmd] -> bus_creator/4  "CAN4_FDC_BCM_FrAtmoLamp_Cmd"
  [CAN4_FDC_BCM_FrRmLampBright_Cmd] -> bus_creator/5  "CAN4_FDC_BCM_FrRmLampBright_Cmd"
  [CAN4_FDC_BCM_FrRoomlamp_Cmd] -> bus_creator/6  "CAN4_FDC_BCM_FrRoomlamp_Cmd"
  [CAN4_FDC_BCM_IBuzzerReq_Sta] -> bus_creator/7  "CAN4_FDC_BCM_IBuzzerReq_Sta"
  [CAN4_FDC_BCM_LSMLP_Cmd] -> bus_creator/8  "CAN4_FDC_BCM_LSMLP_Cmd"
  [CAN4_FDC_BCM_LTgateRel_Cmd] -> bus_creator/9  "CAN4_FDC_BCM_LTgateRel_Cmd"
  [CAN4_FDC_BCM_RSMLP_Cmd] -> bus_creator/10  "CAN4_FDC_BCM_RSMLP_Cmd"
  [CAN4_FDC_BCM_RTgateRel_Cmd] -> bus_creator/11  "CAN4_FDC_BCM_RTgateRel_Cmd"
  [CAN4_FDC_BCM_RevBuzzerout_Cmd] -> bus_creator/12  "CAN4_FDC_BCM_RevBuzzerout_Cmd"
  [CAN4_FDC_BCM_RrAtmoLamp_Cmd] -> bus_creator/13  "CAN4_FDC_BCM_RrAtmoLamp_Cmd"
  [CAN4_FDC_BCM_RrRmLampBright_Cmd] -> bus_creator/14  "CAN4_FDC_BCM_RrRmLampBright_Cmd"
  [CAN4_FDC_BCM_RrRoomlamp_Cmd] -> bus_creator/15  "CAN4_FDC_BCM_RrRoomlamp_Cmd"
  [CAN4_FDC_BCM_STurnLpLeft_Cmd] -> bus_creator/16  "CAN4_FDC_BCM_STurnLpLeft_Cmd"
  [CAN4_FDC_BCM_STurnLpRight_Cmd] -> bus_creator/17  "CAN4_FDC_BCM_STurnLpRight_Cmd"
  [CAN4_FDC_BCM_TgateHDSWL_Sta] -> bus_creator/18  "CAN4_FDC_BCM_TgateHDSWL_Sta"
  [CAN4_FDC_BCM_TgateHDSWR_Sta] -> bus_creator/19  "CAN4_FDC_BCM_TgateHDSWR_Sta"
  [CAN4_FDC_BCM_TgateSWL_Sta] -> bus_creator/20  "CAN4_FDC_BCM_TgateSWL_Sta"
  [CAN4_FDC_BCM_TgateSWR_Sta] -> bus_creator/21  "CAN4_FDC_BCM_TgateSWR_Sta"
  [CAN4_FDC_BCM_TurnLpLActive_Cmd] -> bus_creator/22  "CAN4_FDC_BCM_TurnLpLActive_Cmd"
  [CAN4_FDC_BCM_TurnLpRActive_Cmd] -> bus_creator/23  "CAN4_FDC_BCM_TurnLpRActive_Cmd"
  [CAN4_FDC_BCM_innerBuzzer_Cmd] -> bus_creator/24  "CAN4_FDC_BCM_innerBuzzer_Cmd"
  bus_creator/1 -> FD4_CE100_3/1
  FDCBCMBBuzzerCmd/1(CAN4_FDC_BCM_BBuzzer_Cmd) -> [CAN4_FDC_BCM_BBuzzer_Cmd]
  FDCBCMBBuzzeroutCmd/1(CAN4_FDC_BCM_BBuzzerout_Cmd) -> [CAN4_FDC_BCM_BBuzzerout_Cmd]
  FDCBCMEmExitLightCmd/1(CAN4_FDC_BCM_EmExitLight_Cmd) -> [CAN4_FDC_BCM_EmExitLight_Cmd]
  FDCBCMFrAtmoLampCmd/1(CAN4_FDC_BCM_FrAtmoLamp_Cmd) -> [CAN4_FDC_BCM_FrAtmoLamp_Cmd]
  FDCBCMFrRmLampBrightCmd/1(CAN4_FDC_BCM_FrRmLampBright_Cmd) -> [CAN4_FDC_BCM_FrRmLampBright_Cmd]
  FDCBCMFrRoomlampCmd/1(CAN4_FDC_BCM_FrRoomlamp_Cmd) -> [CAN4_FDC_BCM_FrRoomlamp_Cmd]
  FDCBCMIBuzzerReqSta/1(CAN4_FDC_BCM_IBuzzerReq_Sta) -> [CAN4_FDC_BCM_IBuzzerReq_Sta]
  FDCBCMLSMLPCmd/1(CAN4_FDC_BCM_LSMLP_Cmd) -> [CAN4_FDC_BCM_LSMLP_Cmd]
  FDCBCMLTgateRelCmd/1(CAN4_FDC_BCM_LTgateRel_Cmd) -> [CAN4_FDC_BCM_LTgateRel_Cmd]
  FDCBCMRSMLPCmd/1(CAN4_FDC_BCM_RSMLP_Cmd) -> [CAN4_FDC_BCM_RSMLP_Cmd]
  FDCBCMRTgateRelCmd/1(CAN4_FDC_BCM_RTgateRel_Cmd) -> [CAN4_FDC_BCM_RTgateRel_Cmd]
  FDCBCMRevBuzzeroutCmd/1(CAN4_FDC_BCM_RevBuzzerout_Cmd) -> [CAN4_FDC_BCM_RevBuzzerout_Cmd]
  FDCBCMRrAtmoLampCmd/1(CAN4_FDC_BCM_RrAtmoLamp_Cmd) -> [CAN4_FDC_BCM_RrAtmoLamp_Cmd]
  FDCBCMRrRmLampBrightCmd/1(CAN4_FDC_BCM_RrRmLampBright_Cmd) -> [CAN4_FDC_BCM_RrRmLampBright_Cmd]
  FDCBCMRrRoomlampCmd/1(CAN4_FDC_BCM_RrRoomlamp_Cmd) -> [CAN4_FDC_BCM_RrRoomlamp_Cmd]
  FDCBCMSTurnLpLeftCmd/1(CAN4_FDC_BCM_STurnLpLeft_Cmd) -> [CAN4_FDC_BCM_STurnLpLeft_Cmd]
  FDCBCMSTurnLpRightCmd/1(CAN4_FDC_BCM_STurnLpRight_Cmd) -> [CAN4_FDC_BCM_STurnLpRight_Cmd]
  FDCBCMTgateHDSWLSta/1(CAN4_FDC_BCM_TgateHDSWL_Sta) -> [CAN4_FDC_BCM_TgateHDSWL_Sta]
  FDCBCMTgateHDSWRSta/1(CAN4_FDC_BCM_TgateHDSWR_Sta) -> [CAN4_FDC_BCM_TgateHDSWR_Sta]
  FDCBCMTgateSWLSta/1(CAN4_FDC_BCM_TgateSWL_Sta) -> [CAN4_FDC_BCM_TgateSWL_Sta]
  FDCBCMTgateSWRSta/1(CAN4_FDC_BCM_TgateSWR_Sta) -> [CAN4_FDC_BCM_TgateSWR_Sta]
  FDCBCMTurnLpLActiveCmd/1(CAN4_FDC_BCM_TurnLpLActive_Cmd) -> [CAN4_FDC_BCM_TurnLpLActive_Cmd]
  FDCBCMTurnLpRActiveCmd/1(CAN4_FDC_BCM_TurnLpRActive_Cmd) -> [CAN4_FDC_BCM_TurnLpRActive_Cmd]
  FDCBCMinnerBuzzerCmd/1(CAN4_FDC_BCM_innerBuzzer_Cmd) -> [CAN4_FDC_BCM_innerBuzzer_Cmd]
  bus_selector/1 -> FDCBCMBBuzzerCmd/1(FDCBCMBBuzzerCmd)  "<VOUTP_BBuzzerCmd_flg>"
  [BOUTP_outputs] -> bus_selector/1
  Ground/1 -> FDCBCMBBuzzeroutCmd/1(FDCBCMBBuzzeroutCmd)
  Ground1/1 -> FDCBCMEmExitLightCmd/1(FDCBCMEmExitLightCmd)
  bus_selector1/1 -> FDCBCMFrAtmoLampCmd/1(FDCBCMFrAtmoLampCmd)  "<VOUTP_FrAtmoLampCmd_flg>"
  [BOUTP_outputs] -> bus_selector1/1
  Ground2/1 -> FDCBCMFrRmLampBrightCmd/1(FDCBCMFrRmLampBrightCmd)
  Ground3/1 -> FDCBCMFrRoomlampCmd/1(FDCBCMFrRoomlampCmd)
  Ground4/1 -> FDCBCMIBuzzerReqSta/1(FDCBCMIBuzzerReqSta)
  bus_selector2/1 -> FDCBCMLSMLPCmd/1(FDCBCMLSMLPCmd)  "<VOUTP_LSMLPCmd_flg>"
  [BOUTP_outputs] -> bus_selector2/1
  bus_selector3/1 -> FDCBCMLTgateRelCmd/1(FDCBCMLTgateRelCmd)  "<VOUTP_LTgateRelCmd_flg>"
  [BOUTP_outputs] -> bus_selector3/1
  bus_selector4/1 -> FDCBCMRSMLPCmd/1(FDCBCMRSMLPCmd)  "<VOUTP_RSMLPCmd_flg>"
  [BOUTP_outputs] -> bus_selector4/1
  bus_selector5/1 -> FDCBCMRTgateRelCmd/1(FDCBCMRTgateRelCmd)  "<VOUTP_RTgateRelCmd_flg>"
  [BOUTP_outputs] -> bus_selector5/1
  Ground5/1 -> FDCBCMRevBuzzeroutCmd/1(FDCBCMRevBuzzeroutCmd)
  bus_selector6/1 -> FDCBCMRrAtmoLampCmd/1(FDCBCMRrAtmoLampCmd)  "<VOUTP_RrAtmoLampCmd_flg>"
  [BOUTP_outputs] -> bus_selector6/1
  bus_selector7/1 -> FDCBCMRrRmLampBrightCmd/1(FDCBCMRrRmLampBrightCmd)  "<VOUTP_RrRmLampBrightCmd_enum>"
  [BOUTP_outputs] -> bus_selector7/1
  Ground6/1 -> FDCBCMRrRoomlampCmd/1(FDCBCMRrRoomlampCmd)
  Ground7/1 -> FDCBCMSTurnLpLeftCmd/1(FDCBCMSTurnLpLeftCmd)
  Ground8/1 -> FDCBCMSTurnLpRightCmd/1(FDCBCMSTurnLpRightCmd)
  bus_selector8/1 -> FDCBCMTgateHDSWLSta/1(FDCBCMTgateHDSWLSta)  "<VOUTP_TgateHDSWLSta_flg>"
  [BOUTP_outputs] -> bus_selector8/1
  bus_selector9/1 -> FDCBCMTgateHDSWRSta/1(FDCBCMTgateHDSWRSta)  "<VOUTP_TgateHDSWRSta_flg>"
  [BOUTP_outputs] -> bus_selector9/1
  bus_selector10/1 -> FDCBCMTgateSWLSta/1(FDCBCMTgateSWLSta)  "<VOUTP_TgateSWLSta_flg>"
  [BOUTP_outputs] -> bus_selector10/1
  bus_selector11/1 -> FDCBCMTgateSWRSta/1(FDCBCMTgateSWRSta)  "<VOUTP_TgateSWRSta_flg>"
  [BOUTP_outputs] -> bus_selector11/1
  bus_selector12/1 -> FDCBCMTurnLpLActiveCmd/1(FDCBCMTurnLpLActiveCmd)  "<VOUTP_TurnLpLActiveCmd_flg>"
  [BOUTP_outputs] -> bus_selector12/1
  bus_selector13/1 -> FDCBCMTurnLpRActiveCmd/1(FDCBCMTurnLpRActiveCmd)  "<VOUTP_TurnLpRActiveCmd_flg>"
  [BOUTP_outputs] -> bus_selector13/1
  Ground9/1 -> FDCBCMinnerBuzzerCmd/1(FDCBCMinnerBuzzerCmd)

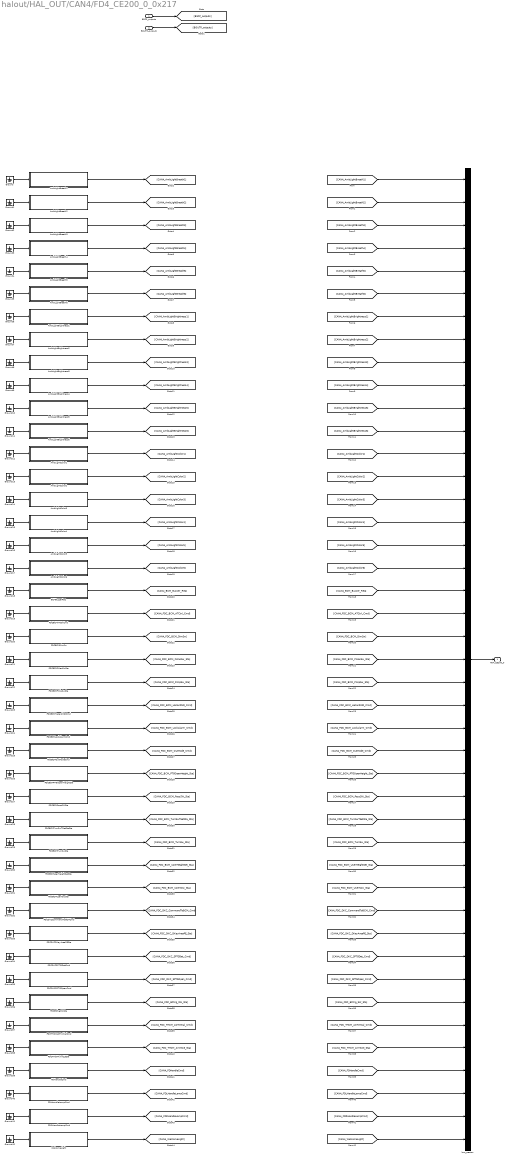
== system halout/HAL_OUT/CAN4/FD4_CE200_0_0x217 ==
  BSCP_outputs : Inport  OutDataTypeStr=Bus: BSCP_outputs
  BOUTP_outputs : Inport  Port=2  OutDataTypeStr=Bus: BOUTP_outputs
  AmbLightBreath1 : Subsystem
  AmbLightBreath2 : Subsystem
  AmbLightBreath3 : Subsystem
  AmbLightBreath4 : Subsystem
  AmbLightBreath5 : Subsystem
  AmbLightBreath6 : Subsystem
  AmbLightBrightness1 : Subsystem
  AmbLightBrightness2 : Subsystem
  AmbLightBrightness3 : Subsystem
  AmbLightBrightness4 : Subsystem
  AmbLightBrightness5 : Subsystem
  AmbLightBrightness6 : Subsystem
  AmbLightColor1 : Subsystem
  AmbLightColor2 : Subsystem
  AmbLightColor3 : Subsystem
  AmbLightColor4 : Subsystem
  AmbLightColor5 : Subsystem
  AmbLightColor6 : Subsystem
  BCMBuzzerReq : Subsystem
  FDCBCMATCtrlCmd : Subsystem
  FDCBCMDimSw : Subsystem
  FDCBCMFWasSwSta : Subsystem
  FDCBCMFWipSwSta : Subsystem
  FDCBCMHazardINDCmd : Subsystem
  FDCBCMLockAlarmCmd : Subsystem
  FDCBCMOutModeCmd : Subsystem
  FDCBCMPTGOpenHeightSta : Subsystem
  FDCBCMPassSWSta : Subsystem
  FDCBCMTurnSwSta : Subsystem
  FDCBCMTurnSwTSetStaSta : Subsystem
  FDCBCMUserHeightSetSta : Subsystem
  FDCBCMUserNowSta : Subsystem
  FDCDKCCommandToBCMCmd : Subsystem
  FDCDKCDKeyAreaPESta : Subsystem
  FDCDKCSPTGDetCmd : Subsystem
  FDCDKCSPTGOpenCmd : Subsystem
  FDCEChrgSWSta : Subsystem
  FDCTHCMACTInitialCmd : Subsystem
  FDCTHCMAirIntZ3Sta : Subsystem
  FDHandleCmd : Subsystem
  FDLHandleLampCmd : Subsystem
  FDRHandleLampCmd : Subsystem
  Ground{,1..42} (43 alike) : Ground
  WelcomeLight : Subsystem
  bus_creator : BusCreator  Inputs=43  OutDataTypeStr=Bus: DT_CAN4_SG_FD4_CE200_0  NonVirtualBus=on
  FD4_CE200_0 : Outport
  wires:
  BSCP_outputs/1 -> [BSCP_outputs]
  BOUTP_outputs/1 -> [BOUTP_outputs]
  [CAN4_AmbLightBreath1] -> bus_creator/1  "CAN4_AmbLightBreath1"
  [CAN4_AmbLightBreath2] -> bus_creator/2  "CAN4_AmbLightBreath2"
  [CAN4_AmbLightBreath3] -> bus_creator/3  "CAN4_AmbLightBreath3"
  [CAN4_AmbLightBreath4] -> bus_creator/4  "CAN4_AmbLightBreath4"
  [CAN4_AmbLightBreath5] -> bus_creator/5  "CAN4_AmbLightBreath5"
  [CAN4_AmbLightBreath6] -> bus_creator/6  "CAN4_AmbLightBreath6"
  [CAN4_AmbLightBrightness1] -> bus_creator/7  "CAN4_AmbLightBrightness1"
  [CAN4_AmbLightBrightness2] -> bus_creator/8  "CAN4_AmbLightBrightness2"
  [CAN4_AmbLightBrightness3] -> bus_creator/9  "CAN4_AmbLightBrightness3"
  [CAN4_AmbLightBrightness4] -> bus_creator/10  "CAN4_AmbLightBrightness4"
  [CAN4_AmbLightBrightness5] -> bus_creator/11  "CAN4_AmbLightBrightness5"
  [CAN4_AmbLightBrightness6] -> bus_creator/12  "CAN4_AmbLightBrightness6"
  [CAN4_AmbLightColor1] -> bus_creator/13  "CAN4_AmbLightColor1"
  [CAN4_AmbLightColor2] -> bus_creator/14  "CAN4_AmbLightColor2"
  [CAN4_AmbLightColor3] -> bus_creator/15  "CAN4_AmbLightColor3"
  [CAN4_AmbLightColor4] -> bus_creator/16  "CAN4_AmbLightColor4"
  [CAN4_AmbLightColor5] -> bus_creator/17  "CAN4_AmbLightColor5"
  [CAN4_AmbLightColor6] -> bus_creator/18  "CAN4_AmbLightColor6"
  [CAN4_BCM_Buzzer_Req] -> bus_creator/19  "CAN4_BCM_Buzzer_Req"
  [CAN4_FDC_BCM_ATCtrl_Cmd] -> bus_creator/20  "CAN4_FDC_BCM_ATCtrl_Cmd"
  [CAN4_FDC_BCM_DimSw] -> bus_creator/21  "CAN4_FDC_BCM_DimSw"
  [CAN4_FDC_BCM_FWasSw_Sta] -> bus_creator/22  "CAN4_FDC_BCM_FWasSw_Sta"
  [CAN4_FDC_BCM_FWipSw_Sta] -> bus_creator/23  "CAN4_FDC_BCM_FWipSw_Sta"
  [CAN4_FDC_BCM_HazardIND_Cmd] -> bus_creator/24  "CAN4_FDC_BCM_HazardIND_Cmd"
  [CAN4_FDC_BCM_LockAlarm_Cmd] -> bus_creator/25  "CAN4_FDC_BCM_LockAlarm_Cmd"
  [CAN4_FDC_BCM_OutMode_Cmd] -> bus_creator/26  "CAN4_FDC_BCM_OutMode_Cmd"
  [CAN4_FDC_BCM_PTGOpenHeight_Sta] -> bus_creator/27  "CAN4_FDC_BCM_PTGOpenHeight_Sta"
  [CAN4_FDC_BCM_PassSW_Sta] -> bus_creator/28  "CAN4_FDC_BCM_PassSW_Sta"
  [CAN4_FDC_BCM_TurnSwTSetSta_Sta] -> bus_creator/29  "CAN4_FDC_BCM_TurnSwTSetSta_Sta"
  [CAN4_FDC_BCM_TurnSw_Sta] -> bus_creator/30  "CAN4_FDC_BCM_TurnSw_Sta"
  [CAN4_FDC_BCM_UserHeightSet_Sta] -> bus_creator/31  "CAN4_FDC_BCM_UserHeightSet_Sta"
  [CAN4_FDC_BCM_UserNow_Sta] -> bus_creator/32  "CAN4_FDC_BCM_UserNow_Sta"
  [CAN4_FDC_DKC_CommandToBCM_Cmd] -> bus_creator/33  "CAN4_FDC_DKC_CommandToBCM_Cmd"
  [CAN4_FDC_DKC_DKeyAreaPE_Sta] -> bus_creator/34  "CAN4_FDC_DKC_DKeyAreaPE_Sta"
  [CAN4_FDC_DKC_SPTGDet_Cmd] -> bus_creator/35  "CAN4_FDC_DKC_SPTGDet_Cmd"
  [CAN4_FDC_DKC_SPTGOpen_Cmd] -> bus_creator/36  "CAN4_FDC_DKC_SPTGOpen_Cmd"
  [CAN4_FDC_EChrg_SW_Sta] -> bus_creator/37  "CAN4_FDC_EChrg_SW_Sta"
  [CAN4_FDC_THCM_ACTInitial_Cmd] -> bus_creator/38  "CAN4_FDC_THCM_ACTInitial_Cmd"
  [CAN4_FDC_THCM_AirIntZ3_Sta] -> bus_creator/39  "CAN4_FDC_THCM_AirIntZ3_Sta"
  [CAN4_FDHandleCmd] -> bus_creator/40  "CAN4_FDHandleCmd"
  [CAN4_FDLHandleLampCmd] -> bus_creator/41  "CAN4_FDLHandleLampCmd"
  [CAN4_FDRHandleLampCmd] -> bus_creator/42  "CAN4_FDRHandleLampCmd"
  [CAN4_WelcomeLight] -> bus_creator/43  "CAN4_WelcomeLight"
  bus_creator/1 -> FD4_CE200_0/1
  AmbLightBreath1/1(CAN4_AmbLightBreath1) -> [CAN4_AmbLightBreath1]
  AmbLightBreath2/1(CAN4_AmbLightBreath2) -> [CAN4_AmbLightBreath2]
  AmbLightBreath3/1(CAN4_AmbLightBreath3) -> [CAN4_AmbLightBreath3]
  AmbLightBreath4/1(CAN4_AmbLightBreath4) -> [CAN4_AmbLightBreath4]
  AmbLightBreath5/1(CAN4_AmbLightBreath5) -> [CAN4_AmbLightBreath5]
  AmbLightBreath6/1(CAN4_AmbLightBreath6) -> [CAN4_AmbLightBreath6]
  AmbLightBrightness1/1(CAN4_AmbLightBrightness1) -> [CAN4_AmbLightBrightness1]
  AmbLightBrightness2/1(CAN4_AmbLightBrightness2) -> [CAN4_AmbLightBrightness2]
  AmbLightBrightness3/1(CAN4_AmbLightBrightness3) -> [CAN4_AmbLightBrightness3]
  AmbLightBrightness4/1(CAN4_AmbLightBrightness4) -> [CAN4_AmbLightBrightness4]
  AmbLightBrightness5/1(CAN4_AmbLightBrightness5) -> [CAN4_AmbLightBrightness5]
  AmbLightBrightness6/1(CAN4_AmbLightBrightness6) -> [CAN4_AmbLightBrightness6]
  AmbLightColor1/1(CAN4_AmbLightColor1) -> [CAN4_AmbLightColor1]
  AmbLightColor2/1(CAN4_AmbLightColor2) -> [CAN4_AmbLightColor2]
  AmbLightColor3/1(CAN4_AmbLightColor3) -> [CAN4_AmbLightColor3]
  AmbLightColor4/1(CAN4_AmbLightColor4) -> [CAN4_AmbLightColor4]
  AmbLightColor5/1(CAN4_AmbLightColor5) -> [CAN4_AmbLightColor5]
  AmbLightColor6/1(CAN4_AmbLightColor6) -> [CAN4_AmbLightColor6]
  BCMBuzzerReq/1(CAN4_BCM_Buzzer_Req) -> [CAN4_BCM_Buzzer_Req]
  FDCBCMATCtrlCmd/1(CAN4_FDC_BCM_ATCtrl_Cmd) -> [CAN4_FDC_BCM_ATCtrl_Cmd]
  FDCBCMDimSw/1(CAN4_FDC_BCM_DimSw) -> [CAN4_FDC_BCM_DimSw]
  FDCBCMFWasSwSta/1(CAN4_FDC_BCM_FWasSw_Sta) -> [CAN4_FDC_BCM_FWasSw_Sta]
  FDCBCMFWipSwSta/1(CAN4_FDC_BCM_FWipSw_Sta) -> [CAN4_FDC_BCM_FWipSw_Sta]
  FDCBCMHazardINDCmd/1(CAN4_FDC_BCM_HazardIND_Cmd) -> [CAN4_FDC_BCM_HazardIND_Cmd]
  FDCBCMLockAlarmCmd/1(CAN4_FDC_BCM_LockAlarm_Cmd) -> [CAN4_FDC_BCM_LockAlarm_Cmd]
  FDCBCMOutModeCmd/1(CAN4_FDC_BCM_OutMode_Cmd) -> [CAN4_FDC_BCM_OutMode_Cmd]
  FDCBCMPTGOpenHeightSta/1(CAN4_FDC_BCM_PTGOpenHeight_Sta) -> [CAN4_FDC_BCM_PTGOpenHeight_Sta]
  FDCBCMPassSWSta/1(CAN4_FDC_BCM_PassSW_Sta) -> [CAN4_FDC_BCM_PassSW_Sta]
  FDCBCMTurnSwTSetStaSta/1(CAN4_FDC_BCM_TurnSwTSetSta_Sta) -> [CAN4_FDC_BCM_TurnSwTSetSta_Sta]
  FDCBCMTurnSwSta/1(CAN4_FDC_BCM_TurnSw_Sta) -> [CAN4_FDC_BCM_TurnSw_Sta]
  FDCBCMUserHeightSetSta/1(CAN4_FDC_BCM_UserHeightSet_Sta) -> [CAN4_FDC_BCM_UserHeightSet_Sta]
  FDCBCMUserNowSta/1(CAN4_FDC_BCM_UserNow_Sta) -> [CAN4_FDC_BCM_UserNow_Sta]
  FDCDKCCommandToBCMCmd/1(CAN4_FDC_DKC_CommandToBCM_Cmd) -> [CAN4_FDC_DKC_CommandToBCM_Cmd]
  FDCDKCDKeyAreaPESta/1(CAN4_FDC_DKC_DKeyAreaPE_Sta) -> [CAN4_FDC_DKC_DKeyAreaPE_Sta]
  FDCDKCSPTGDetCmd/1(CAN4_FDC_DKC_SPTGDet_Cmd) -> [CAN4_FDC_DKC_SPTGDet_Cmd]
  FDCDKCSPTGOpenCmd/1(CAN4_FDC_DKC_SPTGOpen_Cmd) -> [CAN4_FDC_DKC_SPTGOpen_Cmd]
  FDCEChrgSWSta/1(CAN4_FDC_EChrg_SW_Sta) -> [CAN4_FDC_EChrg_SW_Sta]
  FDCTHCMACTInitialCmd/1(CAN4_FDC_THCM_ACTInitial_Cmd) -> [CAN4_FDC_THCM_ACTInitial_Cmd]
  FDCTHCMAirIntZ3Sta/1(CAN4_FDC_THCM_AirIntZ3_Sta) -> [CAN4_FDC_THCM_AirIntZ3_Sta]
  FDHandleCmd/1(CAN4_FDHandleCmd) -> [CAN4_FDHandleCmd]
  FDLHandleLampCmd/1(CAN4_FDLHandleLampCmd) -> [CAN4_FDLHandleLampCmd]
  FDRHandleLampCmd/1(CAN4_FDRHandleLampCmd) -> [CAN4_FDRHandleLampCmd]
  WelcomeLight/1(CAN4_WelcomeLight) -> [CAN4_WelcomeLight]
  Ground/1 -> AmbLightBreath1/1(AmbLightBreath1)
  Ground1/1 -> AmbLightBreath2/1(AmbLightBreath2)
  Ground2/1 -> AmbLightBreath3/1(AmbLightBreath3)
  Ground3/1 -> AmbLightBreath4/1(AmbLightBreath4)
  Ground4/1 -> AmbLightBreath5/1(AmbLightBreath5)
  Ground5/1 -> AmbLightBreath6/1(AmbLightBreath6)
  Ground6/1 -> AmbLightBrightness1/1(AmbLightBrightness1)
  Ground7/1 -> AmbLightBrightness2/1(AmbLightBrightness2)
  Ground8/1 -> AmbLightBrightness3/1(AmbLightBrightness3)
  Ground9/1 -> AmbLightBrightness4/1(AmbLightBrightness4)
  Ground10/1 -> AmbLightBrightness5/1(AmbLightBrightness5)
  Ground11/1 -> AmbLightBrightness6/1(AmbLightBrightness6)
  Ground12/1 -> AmbLightColor1/1(AmbLightColor1)
  Ground13/1 -> AmbLightColor2/1(AmbLightColor2)
  Ground14/1 -> AmbLightColor3/1(AmbLightColor3)
  Ground15/1 -> AmbLightColor4/1(AmbLightColor4)
  Ground16/1 -> AmbLightColor5/1(AmbLightColor5)
  Ground17/1 -> AmbLightColor6/1(AmbLightColor6)
  Ground18/1 -> BCMBuzzerReq/1(BCMBuzzerReq)
  Ground19/1 -> FDCBCMATCtrlCmd/1(FDCBCMATCtrlCmd)
  Ground20/1 -> FDCBCMDimSw/1(FDCBCMDimSw)
  Ground21/1 -> FDCBCMFWasSwSta/1(FDCBCMFWasSwSta)
  Ground22/1 -> FDCBCMFWipSwSta/1(FDCBCMFWipSwSta)
  Ground23/1 -> FDCBCMHazardINDCmd/1(FDCBCMHazardINDCmd)
  Ground24/1 -> FDCBCMLockAlarmCmd/1(FDCBCMLockAlarmCmd)
  Ground25/1 -> FDCBCMOutModeCmd/1(FDCBCMOutModeCmd)
  Ground26/1 -> FDCBCMPTGOpenHeightSta/1(FDCBCMPTGOpenHeightSta)
  Ground27/1 -> FDCBCMPassSWSta/1(FDCBCMPassSWSta)
  Ground28/1 -> FDCBCMTurnSwTSetStaSta/1(FDCBCMTurnSwTSetStaSta)
  Ground29/1 -> FDCBCMTurnSwSta/1(FDCBCMTurnSwSta)
  Ground30/1 -> FDCBCMUserHeightSetSta/1(FDCBCMUserHeightSetSta)
  Ground31/1 -> FDCBCMUserNowSta/1(FDCBCMUserNowSta)
  Ground32/1 -> FDCDKCCommandToBCMCmd/1(FDCDKCCommandToBCMCmd)
  Ground33/1 -> FDCDKCDKeyAreaPESta/1(FDCDKCDKeyAreaPESta)
  Ground34/1 -> FDCDKCSPTGDetCmd/1(FDCDKCSPTGDetCmd)
  Ground35/1 -> FDCDKCSPTGOpenCmd/1(FDCDKCSPTGOpenCmd)
  Ground36/1 -> FDCEChrgSWSta/1(FDCEChrgSWSta)
  Ground37/1 -> FDCTHCMACTInitialCmd/1(FDCTHCMACTInitialCmd)
  Ground38/1 -> FDCTHCMAirIntZ3Sta/1(FDCTHCMAirIntZ3Sta)
  Ground39/1 -> FDHandleCmd/1(FDHandleCmd)
  Ground40/1 -> FDLHandleLampCmd/1(FDLHandleLampCmd)
  Ground41/1 -> FDRHandleLampCmd/1(FDRHandleLampCmd)
  Ground42/1 -> WelcomeLight/1(WelcomeLight)

== system halout/HAL_OUT/CAN4/Function-Call Subsystem ==
  function : TriggerPort  TriggerType=function-call  VariantControl=(inherit)
  Add : Sum
  Constant : Constant  Value=ONE_INT
  Constant1 : Constant  Value=ZERO_INT
  Constant2 : Constant  Value=uint8(10)
  GreaterThan : RelationalOperator  Operator=>  OutDataTypeStr=boolean  RndMeth=Simplest
  Switch : Switch  Criteria=u2 ~= 0
  Unit Delay : UnitDelay  SampleTime=-1  HasFrameUpgradeWarning=on
  TriggerCAN4VCU1_CNT : Outport
  wires:
  Constant1/1 -> Switch/1
  GreaterThan/1 -> Switch/2
  Constant2/1 -> GreaterThan/2
  Switch/1 -> Unit Delay/1, TriggerCAN4VCU1_CNT/1
  Constant/1 -> Add/2
  Unit Delay/1 -> Add/1
  Add/1 -> GreaterThan/1, Switch/3

== system halout/HAL_OUT/CAN4/GW4_CE100_0_0x253 ==
  BSCP_outputs : Inport  OutDataTypeStr=Bus: BSCP_outputs
  BOUTP_outputs : Inport  Port=2  OutDataTypeStr=Bus: BOUTP_outputs
  BrkPedalPos : Subsystem
  BrkPedalPosSta : Subsystem
  BrkSwSta : Subsystem
  BrkSwV : Subsystem
  FDCPTGinnerSW2 : Subsystem
  Ground{,1..8} (9 alike) : Ground
  LDrvCtrlCmd : Subsystem
  LPasCtrlCmd : Subsystem
  LRLDCtrlCmd : Subsystem
  LRRDCtrlCmd : Subsystem
  MCPressure : Subsystem
  MCPressureV : Subsystem
  VehSpeed : Subsystem
  bus_creator : BusCreator  Inputs=12  OutDataTypeStr=Bus: DT_CAN4_SG_GW4_CE100_0  NonVirtualBus=on
  bus_selector : BusSelector  OutputSignals=VOUTP_BrkPedalPos_pct
  bus_selector1 : BusSelector  OutputSignals=VOUTP_SCPBrkSwSta_flg
  bus_selector2 : BusSelector  OutputSignals=VOUTP_Vehspeed_kph
  GW4_CE100_0 : Outport
  wires:
  BSCP_outputs/1 -> [BSCP_outputs]
  BOUTP_outputs/1 -> [BOUTP_outputs]
  [CAN4_BrkPedalPos] -> bus_creator/1  "CAN4_BrkPedalPos"
  [CAN4_BrkPedalPos_Sta] -> bus_creator/2  "CAN4_BrkPedalPos_Sta"
  [CAN4_BrkSw_Sta] -> bus_creator/3  "CAN4_BrkSw_Sta"
  [CAN4_BrkSw_V] -> bus_creator/4  "CAN4_BrkSw_V"
  [CAN4_FDC_PTG_inner_SW_2] -> bus_creator/5  "CAN4_FDC_PTG_inner_SW_2"
  [CAN4_L_Drv_CtrlCmd] -> bus_creator/6  "CAN4_L_Drv_CtrlCmd"
  [CAN4_L_Pas_CtrlCmd] -> bus_creator/7  "CAN4_L_Pas_CtrlCmd"
  [CAN4_L_RLD_CtrlCmd] -> bus_creator/8  "CAN4_L_RLD_CtrlCmd"
  [CAN4_L_RRD_CtrlCmd] -> bus_creator/9  "CAN4_L_RRD_CtrlCmd"
  [CAN4_MCPressure] -> bus_creator/10  "CAN4_MCPressure"
  [CAN4_MCPressure_V] -> bus_creator/11  "CAN4_MCPressure_V"
  [CAN4_VehSpeed] -> bus_creator/12  "CAN4_VehSpeed"
  bus_creator/1 -> GW4_CE100_0/1
  BrkPedalPos/1(CAN4_BrkPedalPos) -> [CAN4_BrkPedalPos]
  BrkPedalPosSta/1(CAN4_BrkPedalPos_Sta) -> [CAN4_BrkPedalPos_Sta]
  BrkSwSta/1(CAN4_BrkSw_Sta) -> [CAN4_BrkSw_Sta]
  BrkSwV/1(CAN4_BrkSw_V) -> [CAN4_BrkSw_V]
  FDCPTGinnerSW2/1(CAN4_FDC_PTG_inner_SW_2) -> [CAN4_FDC_PTG_inner_SW_2]
  LDrvCtrlCmd/1(CAN4_L_Drv_CtrlCmd) -> [CAN4_L_Drv_CtrlCmd]
  LPasCtrlCmd/1(CAN4_L_Pas_CtrlCmd) -> [CAN4_L_Pas_CtrlCmd]
  LRLDCtrlCmd/1(CAN4_L_RLD_CtrlCmd) -> [CAN4_L_RLD_CtrlCmd]
  LRRDCtrlCmd/1(CAN4_L_RRD_CtrlCmd) -> [CAN4_L_RRD_CtrlCmd]
  MCPressure/1(CAN4_MCPressure) -> [CAN4_MCPressure]
  MCPressureV/1(CAN4_MCPressure_V) -> [CAN4_MCPressure_V]
  VehSpeed/1(CAN4_VehSpeed) -> [CAN4_VehSpeed]
  bus_selector/1 -> BrkPedalPos/1(BrkPedalPos)  "<VOUTP_BrkPedalPos_pct>"
  [BOUTP_outputs] -> bus_selector/1
  Ground/1 -> BrkPedalPosSta/1(BrkPedalPosSta)
  bus_selector1/1 -> BrkSwSta/1(BrkSwSta)  "<VOUTP_SCPBrkSwSta_flg>"
  [BOUTP_outputs] -> bus_selector1/1
  Ground1/1 -> BrkSwV/1(BrkSwV)
  Ground2/1 -> FDCPTGinnerSW2/1(FDCPTGinnerSW2)
  Ground3/1 -> LDrvCtrlCmd/1(LDrvCtrlCmd)
  Ground4/1 -> LPasCtrlCmd/1(LPasCtrlCmd)
  Ground5/1 -> LRLDCtrlCmd/1(LRLDCtrlCmd)
  Ground6/1 -> LRRDCtrlCmd/1(LRRDCtrlCmd)
  Ground7/1 -> MCPressure/1(MCPressure)
  Ground8/1 -> MCPressureV/1(MCPressureV)
  bus_selector2/1 -> VehSpeed/1(VehSpeed)  "<VOUTP_Vehspeed_kph>"
  [BOUTP_outputs] -> bus_selector2/1
